simulink model "simulink01"  (R2023b)
settings: Solver=FixedStepAuto  StartTime=0.0  StopTime=0.5  FixedStep=1e-4  RelTol=1e-3
settings Model: Creator=asus  LastModifiedBy=asus

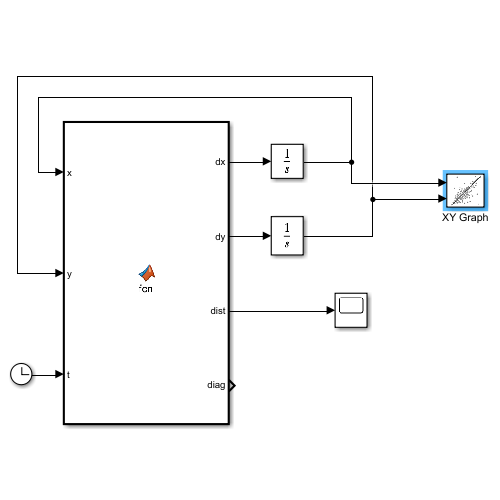
[thumbnail: Simulink's stored preview of the top-level diagram]
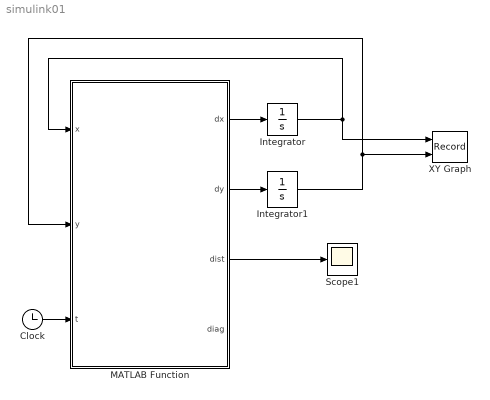
== system simulink01 ==
  Clock : Clock
  Integrator : Integrator
  Integrator1 : Integrator
  MATLAB Function : MATLAB Function  TreatAsAtomicUnit=on
  Scope1 : Scope
  XY Graph : Record  FileSettingsInternal="{\"entries\":[{\"content\":{\"excelSettings\":{\"content\":{},\"type\":\"Streamout.ExcelSettings\"}},\"type\":\"Streamout.FileSettingStorage\",\"uuid\":\"\"}],\"packageUris\":[\"http:\\/\\/schema.mathworks.com\\/mf0\\/streamout_blocks\\/R2020a\"],\"version\":\"1.0\"}"  Layout=[1 1]  SignalsInternal="{\"entries\":[{\"content\":{\"signals\":[{\"content\":{\"blockPath\":[],\"dimensions\":[1],\"domain\":\"\",\"lineColor\":\"#a2142f\",\"plots\":[1],\"port\":1,\"sid\":[\"\"],\"signalID\":258,\"signalName\":\"Integrator\"},\"type\":\"RecordBlkView.Signal\",\"uuid\":\"\"},{\"content\":{\"blockPath\":[],\"dimensions\":[1],\"domain\":\"\",\"lineColor\":\"#139fff\",\"plots\":[1],\"port\":2,\"sid\":[\"\"],\"signalID\":262,\"signalName\":\"Integrator1\"},\"type\":\"RecordBlkView.Signal\",\"uuid\":\"\"}]},\"type\":\"RecordBlkView.InputSignals\",\"uuid\":\"\"}],\"packageUris\":[\"http:\\/\\/schema.mathworks.com\\/mf0\\/streamout_blocks\\/R2020a\"],\"version\":\"1.0\"}"  VisualizationBindings="{\"xyplotplugin\":{\"info\":[{\"series\":[{\"bindingParametersList\":[{\"parameter\":\"X-Axis\",\"signalID\":258,\"signalName\":\"Integrator\"},{\"parameter\":\"Y-Axis\",\"signalID\":262,\"signalName\":\"Integrator1\"}],\"seriesID\":6155}],\"subplotID\":1}]}}"  CompatibilityTag=XY
  wires:
  MATLAB Function/1(dx) -> Integrator/1
  Integrator/1 -> XY Graph/1, MATLAB Function/1(x)
  MATLAB Function/2(dy) -> Integrator1/1
  Integrator1/1 -> XY Graph/2, MATLAB Function/2(y)
  Clock/1 -> MATLAB Function/3(t)
  MATLAB Function/3(dist) -> Scope1/1

== matlab function simulink01/MATLAB Function ==
  data: x input; dx output; y input; t input; dy output; dist output; diag output
function [dx,dy,dist,diag] = fcn(x,y,t)

dist = sqrt( (1 - x)^2 + (t - y)^2 );

if(dist > 0)
    dx = 5 * (1 - x) / dist;
    dy = 5 * (t - y) / dist;
    diag = 0;
elseif(dist == 0)
    dx=0;
    dy=0;
    diag = 1;
else
    dx=0;
    dy=0;
    diag = 2;
end
